simulink model "rigParallelPort"  (R2012b)
settings: Solver=FixedStepDiscrete  SolverMode=MultiTasking  StartTime=0.0  StopTime=10.0  FixedStep=0.001  RelTol=1e-3
undefined symbols (not defined in the file): blockNumber, pause
libraries: xpcparallelportlib x1, simulink x1
settings Model: xpc_rtwmakecfg_data=_xpcetherlib__xpcether8255xlib__xpcetherGbElib__xpcnblib_  BufferReuse=off  Creator=gilja  LastModifiedBy=Chethan
settings SolverCC: EnableConcurrentExecution=on  ConcurrentTasks=on
settings DataIOCC: SaveOutput=off  SignalLogging=off  DSMLogging=off  SaveTime=off
settings OptimizationCC: BlockReduction=off  InlineParams=on  InlineInvariantSignals=on  OptimizeBlockIOStorage=off  BufferReuse=off  ExpressionFolding=off  LocalBlockOutputs=off
settings HardwareCC: ProdIntDivRoundTo=Zero  ProdEndianess=LittleEndian  ProdHWDeviceType=Generic->32-bit x86 compatible
settings ModelReferenceCC: ModelReferenceNumInstancesAllowed=Single  PropagateVarSize=During execution  ModelReferenceMinAlgLoopOccurrences=on
settings RTWCC: SystemTargetFile=xpctarget.tlc  TemplateMakefile=xpc_default_tmf  Description=xPC Target  ProcessScript=xpctarget_make_rtw_hook  RTWCompilerOptimization=On
settings CodeAppCC: MaxIdLength=62
settings xpcTargetCC: TargetFcnLib=ansi_tfl_table_tmw.mat  CodeReplacementLibrary=XPC_BLAS  ParMdlRefBuildCompliant=on  ConcurrentExecutionCompliant=on  CombineSignalStateStructs=off  GRTInterface=on  xPCTaskExecutionProfile=on  xPCRL32EventNumber=5000  xPCisDownloadable=off  xPCLoadParamSetFile=off  xPCConcurrentTasks=off  xPCEnableSFAnimation=off

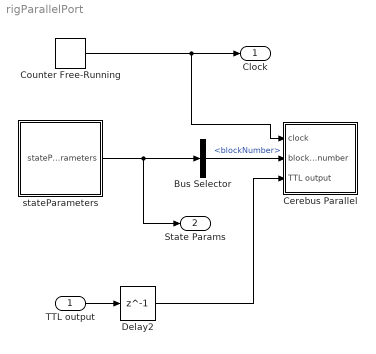
== system rigParallelPort ==
  TTL output : Inport
  Bus Selector : BusSelector  OutputSignals=blockNumber
  Cerebus Parallel : Subsystem
  Counter Free-Running : simulink/Sources/Counter Free-Running  NumBits=32  tsamp=-1
  Delay2 : Delay  DelayLength=1
  stateParameters : Subsystem
  Clock : Outport  OutDataTypeStr=uint32
  State Params : Outport  Port=2  OutDataTypeStr=Bus: stateParams  BusOutputAsStruct=on
  wires:
  stateParameters/1(stateParameters) -> Bus Selector/1, State Params/1
  Counter Free-Running/1 -> Clock/1, Cerebus Parallel/1(clock)
  Bus Selector/1 -> Cerebus Parallel/2(block number)  "<blockNumber>"
  TTL output/1 -> Delay2/1
  Delay2/1 -> Cerebus Parallel/3(TTL output)

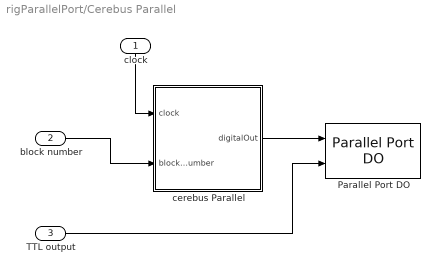
== system rigParallelPort/Cerebus Parallel ==
  clock : Inport
  block number : Inport  Port=2
  TTL output : Inport  Port=3
  "Parallel Port DO " : xpcparallelportlib/Digital Output/Parallel Port DO   BaseMask=0x378  BaseString=0x378  Format=8 1-bit Channels  Channels=[1 2]  InitialValues=[0 0]  FinalActions=[0 0]  FinalValues=[0 0]  SampleTime=0.001  Mode=1
  cerebus Parallel : MATLAB Function  TreatAsAtomicUnit=on
  wires:
  block number/1 -> cerebus Parallel/2(blockNumber)
  clock/1 -> cerebus Parallel/1(clock)
  cerebus Parallel/1(digitalOut) -> "Parallel Port DO "/1
  TTL output/1 -> "Parallel Port DO "/2

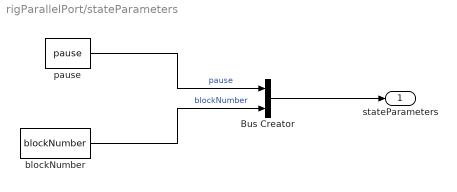
== system rigParallelPort/stateParameters ==
  Bus Creator : BusCreator  Inputs='pause','blockNumber'  OutDataTypeStr=Bus: stateParams  NonVirtualBus=on
  blockNumber : Constant  Value=blockNumber  OutDataTypeStr=uint32
  pause : Constant  Value=pause  OutDataTypeStr=boolean
  stateParameters : Outport
  wires:
  pause/1 -> Bus Creator/1  "pause"
  Bus Creator/1 -> stateParameters/1
  blockNumber/1 -> Bus Creator/2  "blockNumber"

== matlab function rigParallelPort/Cerebus Parallel/cerebus Parallel ==
  data: clock input uint32 size=1; digitalOut output double size=1; blockNumber input uint32 size=1
function digitalOut = digitalCerebusData(clock, blockNumber)
%#codegen
persistent digitalFrame

zeroOne = uint32(1431655765); % the bits of this number alternate between 0 and 1

if(isempty(digitalFrame))
    digitalFrame = uint32([zeroOne zeroOne uint32(blockNumber) uint32(clock) zeroOne zeroOne]);
end

frameLengthBits = 32*length(digitalFrame); % number of bits in the frame

bitPosition = mod(clock, frameLengthBits); % what position are we in for frame output

if(bitPosition==0) % if we are position zero, setup a new frame
    digitalFrame = uint32([zeroOne zeroOne blockNumber clock zeroOne zeroOne]);
end


arrayPosition = floor(double(bitPosition)/32) + 1; % which int32 of the frame are we outputting?
outputInteger = digitalFrame(arrayPosition);

digitalOut = double( bitget(outputInteger, mod(bitPosition,32) + 1) ); % which bit of that int32?
